simulink model "model_v1"  (R2016a)
settings: Solver=VariableStepAuto  StartTime=0.0  StopTime=10.0  RelTol=1e-3
model workspace: external: MATLAB File D:\Ortix\Documents\GitHub\control-system-lab\nick\matlab\params.m (data not in the file)
settings Model: Creator=Ortix  LastModifiedBy=Ortix

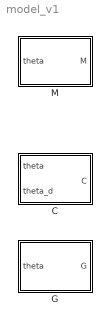
== system model_v1 ==
  C : MATLAB Function  TreatAsAtomicUnit=on
  G : MATLAB Function  TreatAsAtomicUnit=on
  M : MATLAB Function  TreatAsAtomicUnit=on

== matlab function model_v1/C ==
  data: theta input; C output; theta_d input
function C = fcn(theta, theta_d)
%#codegen

C = [b1 - p3*theta_d(2)*sin(theta(2))   -p3*(theta_d(1)+theta_d(2))*sin(theta(2))
    p3*theta_d(1)*sin(theta(2))          b2];

== matlab function model_v1/M ==
  data: theta input; M output
function M = fcn(theta)
%#codegen

M = [p1+p2+2*p3*cos(theta(2))   p2+p3*cos(theta(2));
    p2+p3*cos(theta(2))         p2];

== matlab function model_v1/G ==
  data: theta input; G output
function G = fcn(theta)
%#codegen

C = [-g1*sin(theta(1))-g2*sin(theta(1)+theta(2));
    g2(sin(theta(1)+theta(2))];
